simulink model "solve_chol_sfun_test_TLC18a"  (R2018a)
settings: Solver=FixedStepAuto  StartTime=0.0  StopTime=1  FixedStep=0.5  RelTol=1e-3
values from neighbouring files (symbols this model uses):
  A = 1*exp(-(x-x').^2/2) + eye(D)*1    [test_TLC.m]
  B = rand(D,1)    [test_TLC.m]
settings Model: SimulationMode=rapid-accelerator  Creator=wout7  LastModifiedBy=wout7
settings OptimizationCC: DefaultParameterBehavior=Inlined  AccelVerboseBuild=on
settings DebuggingCC: LibraryContextMissingDiagnostic=warning
settings SFSimCC: SimUserIncludeDirs="\"C:\\Program Files\\MATLAB\\R2018b\\extern\\lib\\win64\\microsoft\\\""  SimUserLibraries=libmwlapack.lib  SimUseLocalCustomCode=on  SimParseCustomCode=off
settings RTWCC: RTWVerbose=off  RetainRTWFile=on  RTWUseLocalCustomCode=on  CustomLibrary=libmwlapack.lib
settings RTWCC: CustomInclude=|
  | "C:\Program Files\MATLAB\R2018b\extern\lib\win64\microsoft\"
  | "C:\Program Files\MATLAB\R2018b\bin\win64\"

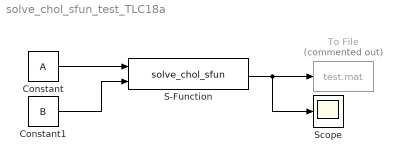
== system solve_chol_sfun_test_TLC18a ==
  Constant : Constant  Value=A
  Constant1 : Constant  Value=B
  S-Function : S-Function  FunctionName=solve_chol_sfun  Parameters=D  SFunctionDeploymentMode=off  EnableBusSupport=off
  Scope : Scope
  To File : ToFile  Commented=on  Filename=test.mat  MatrixName=out
  wires:
  Constant/1 -> S-Function/1
  Constant1/1 -> S-Function/2
  S-Function/1 -> Scope/1, To File/1
